simulink model "STH_Discreto"  (R2020b)
settings: Solver=FixedStepAuto  StartTime=0.0  StopTime=1800  FixedStep=5  RelTol=1e-3
values from neighbouring files (symbols this model uses):
  A = [A11, A12; A21, A22]    [Exp2_STH.m]
  B = horzcat(Bu, Bd)    [Exp2_STH.m]
  C = [1, 0]    [Exp2_STH.m]
  D = [0, 0, 0, 0]    [Exp2_STH.m]
  Gdisc1 = c2d(Gss, 50, 'zoh')    [Exp2_STH.m]
  Gdisc2 = c2d(Gss, 150, 'zoh')    [Exp2_STH.m]
  Gdisc3 = c2d(Gss, 300, 'zoh')    [Exp2_STH.m]
  Ts = 51.67    [Exp2_STH.m]
settings Model: Creator=franc  LastModifiedBy=franc

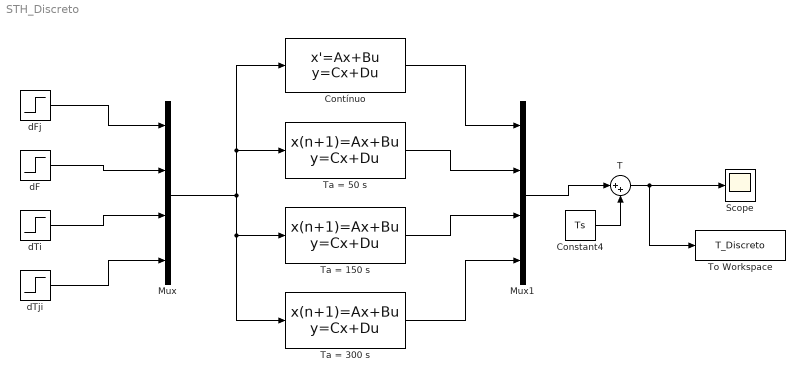
== system STH_Discreto ==
  "            T" : Sum  Inputs=|++
  Constant4 : Constant  Value=Ts
  Contínuo : StateSpace  A=A  B=B  C=C  D=D  InitialCondition=0
  Mux : Mux
  Mux1 : Mux
  Scope : Scope
  Ta = 150 s : DiscreteStateSpace  A=Gdisc2.A  B=Gdisc2.B  C=Gdisc2.C  D=Gdisc2.D  SampleTime=150
  Ta = 300 s : DiscreteStateSpace  A=Gdisc3.A  B=Gdisc3.B  C=Gdisc3.C  D=Gdisc3.D  SampleTime=300
  Ta = 50 s : DiscreteStateSpace  A=Gdisc1.A  B=Gdisc1.B  C=Gdisc1.C  D=Gdisc1.D  SampleTime=50
  To Workspace : ToWorkspace  VariableName=T_Discreto  SaveFormat=Timeseries  SampleTime=-1
  dF : Step  Time=0  After=0  SampleTime=0
  dFj : Step  Time=0  After=4.72e-5  SampleTime=0
  dTi : Step  Time=0  After=0  SampleTime=0
  dTji : Step  Time=0  After=0  SampleTime=0
  wires:
  dTi/1 -> Mux/3
  dFj/1 -> Mux/1
  dTji/1 -> Mux/4
  Mux/1 -> Contínuo/1, Ta = 50 s/1, Ta = 150 s/1, Ta = 300 s/1
  dF/1 -> Mux/2
  Constant4/1 -> "            T"/2
  "            T"/1 -> Scope/1, To Workspace/1
  Ta = 50 s/1 -> Mux1/2
  Contínuo/1 -> Mux1/1
  Mux1/1 -> "            T"/1
  Ta = 150 s/1 -> Mux1/3
  Ta = 300 s/1 -> Mux1/4
